simulink model "cascade_process"  (Simulink 3.00)
libraries: modellib x2

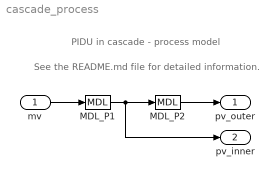
== system cascade_process ==
  note: See the README.md file for detailed information.
  note: PIDU in cascade - process model
  mv : Inport  Port=1
  MDL_P1 : modellib/MDL  k0=100  del=0  tau1=3  tau2=5  nmax=100
  MDL_P2 : modellib/MDL  k0=1  del=0  tau1=3  tau2=5  nmax=100
  pv_outer : Outport  Port=1  nmax=100
  pv_inner : Outport  Port=2  nmax=100
  wires:
  MDL_P1/1 -> MDL_P2/1, pv_inner/1
  MDL_P2/1 -> pv_outer/1
  mv/1 -> MDL_P1/1
